simulink model "MECROKA_TWR_B"  (R2017b)
settings: Solver=FixedStepDiscrete  StartTime=0.0  StopTime=inf  RelTol=1e-3  EnableMultiTasking=on
InitFcn:
  | % BLDC-data
  | num_pol_pairs = 7
  | res_period = 5000;
  | res_pwm   = 2^8;
  | 
  | wheel_radius=0.033;
  | axle_length=0.2;
undefined symbols (not defined in the file): DiscIntNeverNeededParam
libraries: MecRoKa_SFunction_Library x18, arduinolib x12, simulink x5, simulink_extras x2
(part 1 of 2)
settings Model: ExtModeTrigDuration=2  Creator=Bitsch  LastModifiedBy=Lenovo
settings DataIOCC: LimitDataPoints=on  InspectSignalLogs=on
settings OptimizationCC: LifeSpan=1  MaxStackSize=64
settings DebuggingCC: UnderspecifiedInitializationDetection=Classic  MergeDetectMultiDrivingBlocksExec=none  ParameterPrecisionLossMsg=none  AllowSymbolicDim=off  SFUnexpectedBacktrackingDiag=warning  SFNoUnconditionalDefaultTransitionDiag=warning  SFExecutionAtInitializationDiag=none
settings HardwareCC: ProdBitPerPointer=32  ProdBitPerSizeT=32  ProdBitPerPtrDiffT=32  ProdLargestAtomicInteger=Long  ProdLargestAtomicFloat=Double  ProdWordSize=32  ProdHWDeviceType=ARM Compatible->ARM Cortex  UseEmbeddedCoderFeatures=off  UseSimulinkCoderFeatures=off
settings ModelReferenceCC: PropagateSignalLabelsOutOfModel=off
settings SFSimCC: MATLABDynamicMemAlloc=off
settings RTWCC: SystemTargetFile=ert.tlc  HardwareBoard=Arduino Due  TLCOptions=-aInlineSetEventsForThisBaseRateFcn=TLC_FALSE -aSuppressMultiTaskScheduler=TLC_FALSE -aRateBasedStepFcn=1  TemplateMakefile=ert_default_tmf  Toolchain=Arduino ARM  BuildConfiguration=Faster Runs
settings CodeAppCC: StateflowObjectComments=on
settings ERTTargetCC: MultiwordLength=2048  ERTCustomFileBanners=off  SupportContinuousTime=on  SupportNonInlinedSFcns=on  RemoveResetFunc=off  ModelStepFunctionPrototypeControlCompliant=off  ConvertIfToSwitch=off  SuppressUnreachableDefaultCases=off
settings ConfigComp: CovMetricSettings=dw  CovHtmlReporting=on  CovSaveCumulativeToWorkspaceVar=on  CovSaveSingleToWorkspaceVar=on  CovExternalEMLEnable=off

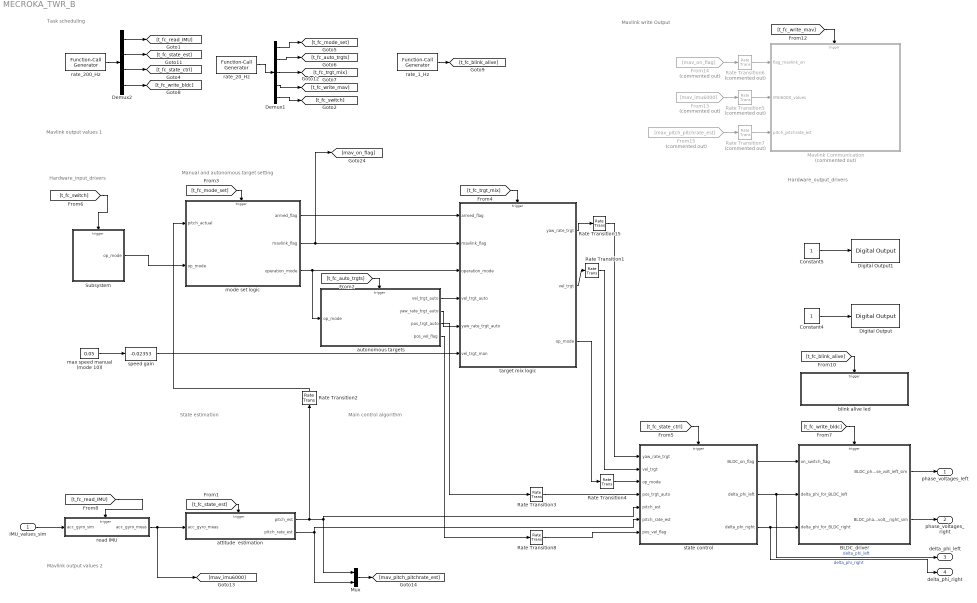
== system MECROKA_TWR_B ==
  note: Mavlink write Output
  note: Mavlink output values 2
  note: Mavlink output values 1
  note: Task scheduling
  note: Manual and autonomous target setting
  note: State estimation
  note: Hardware_output_drivers
  note: Hardware_input_drivers
  note: Main control algorithm
  IMU_values_sim : Inport  OutDataTypeStr=int32  PortDimensions=6
  BLDC_driver : Subsystem  TreatAsAtomicUnit=on
  Constant4 : Constant
  Constant5 : Constant
  Demux1 : Demux  Outputs=5
  Demux2 : Demux
  Digital Output : arduinolib/Digital Output  pinNumber=22  blockPlatform=arduino
  Digital Output1 : arduinolib/Digital Output  pinNumber=24  blockPlatform=arduino
  From13 : From  Commented=on  GotoTag=mav_imu6000
  From14 : From  Commented=on  GotoTag=mav_on_flag
  From15 : From  Commented=on  GotoTag=mav_pitch_pitchrate_est
  Mavlink Communication : Stateflow chart  Commented=on  TreatAsAtomicUnit=on
  Mux : Mux  Inputs=2
  Rate Transition{1..4,8,15} (6 alike) : RateTransition  OutPortSampleTimeOpt=Inherit  OutPortSampleTime=0.01
  Rate Transition5 : RateTransition  Commented=on  OutPortSampleTimeOpt=Inherit  OutPortSampleTime=0.01
  Rate Transition6 : RateTransition  Commented=on  OutPortSampleTimeOpt=Inherit  OutPortSampleTime=0.01
  Rate Transition7 : RateTransition  Commented=on  OutPortSampleTimeOpt=Inherit  OutPortSampleTime=0.01
  Subsystem : Subsystem
  attitude  estimation : Stateflow chart  TreatAsAtomicUnit=on
  autonomous targets : Stateflow chart  TreatAsAtomicUnit=on
  blink alive led : Subsystem  TreatAsAtomicUnit=on
  max speed manual (mode 10)l : Constant  Value=0.05  OutDataTypeStr=double
  mode set logic : Stateflow chart  TreatAsAtomicUnit=on
  rate_1_Hz : simulink/Ports & Subsystems/Function-Call Generator  sample_time=1  numberOfIterations=1
  rate_200_Hz : simulink/Ports & Subsystems/Function-Call Generator  sample_time=0.005  numberOfIterations=1
  rate_20_Hz : simulink/Ports & Subsystems/Function-Call Generator  sample_time=0.05  numberOfIterations=1
  read IMU : Subsystem  TreatAsAtomicUnit=on
  speed gain : simulink/Math Operations/Slider Gain  gain=-0.02353  low=-1  high=1
  state control : Stateflow chart  TreatAsAtomicUnit=on
  target mix logic : Stateflow chart  TreatAsAtomicUnit=on
  phase_voltages_left : Outport
  phase_voltages_right : Outport  Port=2
  delta_phi_left : Outport  Port=3  OutDataTypeStr=double
  delta_phi_right : Outport  Port=4  OutDataTypeStr=double
  wires:
  rate_1_Hz/1 -> [t_fc_blink_alive]
  Rate Transition4/1 -> state control/3(op_mode)
  rate_200_Hz/1 -> Demux2/1
  mode set logic/1(armed_flag) -> target mix logic/1(armed_flag)
  [t_fc_auto_trgts] -> autonomous targets/Trigger
  [t_fc_read_IMU] -> read IMU/Trigger
  Demux2/3 -> [t_fc_state_ctrl]
  rate_20_Hz/1 -> Demux1/1
  target mix logic/3(op_mode) -> Rate Transition4/1
  Demux2/2 -> [t_fc_state_est]
  Rate Transition15/1 -> state control/1(yaw_rate_trgt)
  attitude  estimation/1(pitch_est) -> Rate Transition2/1, Mux/1, state control/5(pitch_est)
  Demux2/1 -> [t_fc_read_IMU]
  [t_fc_state_est] -> attitude  estimation/Trigger
  mode set logic/3(operation_mode) -> autonomous targets/1(op_mode), target mix logic/3(operation_mode)
  [t_fc_state_ctrl] -> state control/Trigger
  Demux2/4 -> [t_fc_write_bldc]
  [t_fc_blink_alive] -> blink alive led/Trigger
  target mix logic/1(yaw_rate_trgt) -> Rate Transition15/1
  target mix logic/2(vel_trgt) -> Rate Transition1/1
  autonomous targets/2(yaw_rate_trgt_auto) -> target mix logic/5(yaw_rate_trgt_auto)
  [t_fc_mode_set] -> mode set logic/Trigger
  read IMU/1(acc_gyro_meas) -> [mav_imu6000], attitude  estimation/1(acc_gyro_meas)
  autonomous targets/1(vel_trgt_auto) -> target mix logic/4(vel_trgt_auto)
  Rate Transition1/1 -> state control/2(vel_trgt)
  IMU_values_sim/1 -> read IMU/1(acc_gyro_sim)
  mode set logic/2(mavlink_flag) -> [mav_on_flag], target mix logic/2(mavlink_flag)
  [t_fc_trgt_mix] -> target mix logic/Trigger
  attitude  estimation/2(pitch_rate_est) -> Mux/2, state control/6(pitch_rate_est)
  [t_fc_write_mav] -> Mavlink Communication/Trigger
  From13/1 -> Rate Transition5/1
  Rate Transition5/1 -> Mavlink Communication/2(IMU6000_values)
  From14/1 -> Rate Transition6/1
  Rate Transition6/1 -> Mavlink Communication/1(flag_mavlink_on)
  Mux/1 -> [mav_pitch_pitchrate_est]
  Rate Transition7/1 -> Mavlink Communication/3(pitch_pitchrate_est)
  From15/1 -> Rate Transition7/1
  state control/2(delta_phi_left) -> delta_phi_left/1, BLDC_driver/2(delta_phi_for_BLDC_left)  "delta_phi_left"
  state control/3(delta_phi_right) -> delta_phi_right/1, BLDC_driver/3(delta_phi_for_BLDC_right)  "delta_phi_right"
  Demux1/1 -> [t_fc_mode_set]
  Demux1/2 -> [t_fc_auto_trgts]
  Demux1/3 -> [t_fc_trgt_mix]
  Demux1/4 -> [t_fc_write_mav]
  [t_fc_write_bldc] -> BLDC_driver/Trigger
  BLDC_driver/1(BLDC_phase_volt_left_sim) -> phase_voltages_left/1
  BLDC_driver/2(BLDC_phase_volt__right_sim) -> phase_voltages_right/1
  speed gain/1 -> target mix logic/6(vel_trgt_man)
  max speed manual (mode 10)l/1 -> speed gain/1
  Rate Transition2/1 -> mode set logic/1(pitch_actual)
  state control/1(BLDC_on_flag) -> BLDC_driver/1(on_switch_flag)
  Constant4/1 -> Digital Output/1
  Constant5/1 -> Digital Output1/1
  autonomous targets/3(pos_trgt_auto) -> Rate Transition3/1
  Rate Transition3/1 -> state control/4(pos_trgt_auto)
  autonomous targets/4(pos_vel_flag) -> Rate Transition8/1
  Rate Transition8/1 -> state control/7(pos_vel_flag)
  Subsystem/1(op_mode) -> mode set logic/2(op_mode)
  Demux1/5 -> [t_fc_switch]
  [t_fc_switch] -> Subsystem/Trigger

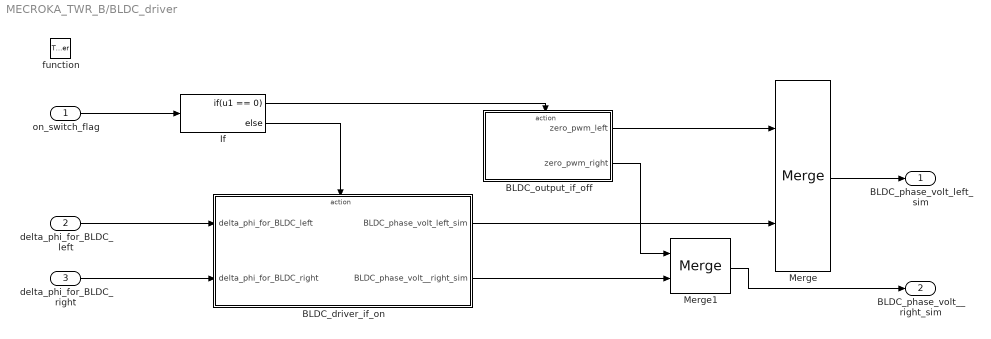
== system MECROKA_TWR_B/BLDC_driver ==
  on_switch_flag : Inport  OutDataTypeStr=boolean  PortDimensions=1
  delta_phi_for_BLDC_left : Inport  Port=2  OutDataTypeStr=double  PortDimensions=1
  delta_phi_for_BLDC_right : Inport  Port=3  OutDataTypeStr=double  PortDimensions=1
  function : TriggerPort  TriggerType=function-call  VariantControl=(inherit)
  BLDC_driver_if_on : Subsystem  TreatAsAtomicUnit=on
  BLDC_output_if_off : Subsystem  TreatAsAtomicUnit=on
  If : If  IfExpression=u1 == 0
  Merge : Merge
  Merge1 : Merge
  BLDC_phase_volt_left_sim : Outport  OutDataTypeStr=uint16  PortDimensions=3
  BLDC_phase_volt__right_sim : Outport  Port=2  OutDataTypeStr=uint16  PortDimensions=3
  wires:
  delta_phi_for_BLDC_right/1 -> BLDC_driver_if_on/2(delta_phi_for_BLDC_right)
  on_switch_flag/1 -> If/1
  BLDC_output_if_off/1(zero_pwm_left) -> Merge/1
  Merge/1 -> BLDC_phase_volt_left_sim/1
  If/1 -> BLDC_output_if_off/Action
  Merge1/1 -> BLDC_phase_volt__right_sim/1
  BLDC_driver_if_on/1(BLDC_phase_volt_left_sim) -> Merge/2
  If/2 -> BLDC_driver_if_on/Action
  BLDC_driver_if_on/2(BLDC_phase_volt__right_sim) -> Merge1/2
  BLDC_output_if_off/2(zero_pwm_right) -> Merge1/1
  delta_phi_for_BLDC_left/1 -> BLDC_driver_if_on/1(delta_phi_for_BLDC_left)

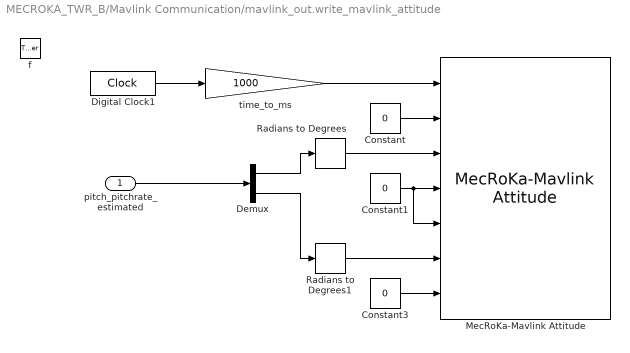
== system MECROKA_TWR_B/Mavlink Communication/mavlink_out.write_mavlink_attitude ==
  pitch_pitchrate_estimated : Inport  OutDataTypeStr=double  PortDimensions=2
  f : TriggerPort  TriggerType=function-call  VariantControl=(inherit)
      settings: CopyFcn=Stateflow.SLINSF.SimulinkMan.removeBlockPreDeleteFcn  PreDeleteFcn=Stateflow.SLINSF.SimulinkMan.unsafePredeleteFcn
  Constant : Constant  Value=0  OutDataTypeStr=double
  Constant1 : Constant  Value=0  OutDataTypeStr=double
  Constant3 : Constant  Value=0  OutDataTypeStr=double
  Demux : Demux  Outputs=2
  Digital Clock1 : DigitalClock  SampleTime=-1
  MecRoKa-Mavlink Attitude : MecRoKa_SFunction_Library/Arduino-Blocks/Mavlink-Library /MecRoKa-Mavlink Attitude  serialPort=0  baudRate=115200  sys_id=2  comp_id=MAV_COMP_ID_ALL
      settings: SourceProductName=MecRoKa_SFunction-Library
  Radians to Degrees : simulink_extras/Transformations/Radians to Degrees
  Radians to Degrees1 : simulink_extras/Transformations/Radians to Degrees
  time_to_ms : Gain  Gain=1000  OutDataTypeStr=uint32
  wires:
  Constant/1 -> MecRoKa-Mavlink Attitude/2
  time_to_ms/1 -> MecRoKa-Mavlink Attitude/1
  Digital Clock1/1 -> time_to_ms/1
  Constant1/1 -> MecRoKa-Mavlink Attitude/5, MecRoKa-Mavlink Attitude/4
  pitch_pitchrate_estimated/1 -> Demux/1
  Demux/1 -> Radians to Degrees/1
  Demux/2 -> Radians to Degrees1/1
  Constant3/1 -> MecRoKa-Mavlink Attitude/7
  Radians to Degrees/1 -> MecRoKa-Mavlink Attitude/3
  Radians to Degrees1/1 -> MecRoKa-Mavlink Attitude/6

== system MECROKA_TWR_B/Mavlink Communication/mavlink_out.write_mavlink_heartbeat ==
  f : TriggerPort  TriggerType=function-call  VariantControl=(inherit)
      settings: CopyFcn=Stateflow.SLINSF.SimulinkMan.removeBlockPreDeleteFcn  PreDeleteFcn=Stateflow.SLINSF.SimulinkMan.unsafePredeleteFcn
  MecRoKa-Mavlink Heartbeat : MecRoKa_SFunction_Library/Arduino-Blocks/Mavlink-Library /MecRoKa-Mavlink Heartbeat  serialPort=0  baudRate=115200  sys_id=2  comp_id=MAV_COMP_ID_ALL  types=MAV_TYPE_GENERIC  autopilot=MAV_AUTOPILOT_GENERIC  base_mode=MAV_MODE_MANUAL_ARMED  custom_mode_m=1  system_status=MAV_STATE_ACTIVE
      settings: SourceProductName=MecRoKa_SFunction-Library

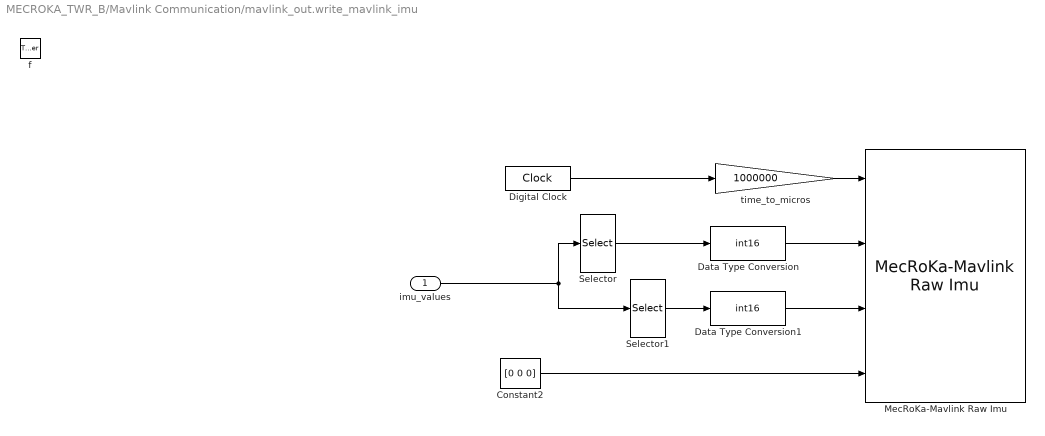
== system MECROKA_TWR_B/Mavlink Communication/mavlink_out.write_mavlink_imu ==
  imu_values : Inport  OutDataTypeStr=int32  PortDimensions=6
  f : TriggerPort  TriggerType=function-call  VariantControl=(inherit)
      settings: CopyFcn=Stateflow.SLINSF.SimulinkMan.removeBlockPreDeleteFcn  PreDeleteFcn=Stateflow.SLINSF.SimulinkMan.unsafePredeleteFcn
  Constant2 : Constant  Value=[0 0 0]  OutDataTypeStr=int16
  Data Type Conversion : DataTypeConversion  OutDataTypeStr=int16
  Data Type Conversion1 : DataTypeConversion  OutDataTypeStr=int16
  Digital Clock : DigitalClock  SampleTime=-1
  MecRoKa-Mavlink Raw Imu : MecRoKa_SFunction_Library/Arduino-Blocks/Mavlink-Library /MecRoKa-Mavlink Raw Imu  serialPort=0  baudRate=115200  sys_id=2  comp_id=MAV_COMP_ID_ALL
      settings: SourceProductName=MecRoKa_SFunction-Library
  Selector : Selector  InputPortWidth=6  IndexOptions=Index vector (dialog)  Indices=[1 2 3]  OutputSizes=1
  Selector1 : Selector  InputPortWidth=6  IndexOptions=Index vector (dialog)  Indices=[4 5 6]  OutputSizes=1
  time_to_micros : Gain  Gain=1000000  OutDataTypeStr=uint32
  wires:
  Data Type Conversion/1 -> MecRoKa-Mavlink Raw Imu/2
  Selector/1 -> Data Type Conversion/1
  Data Type Conversion1/1 -> MecRoKa-Mavlink Raw Imu/3
  Selector1/1 -> Data Type Conversion1/1
  Constant2/1 -> MecRoKa-Mavlink Raw Imu/4
  time_to_micros/1 -> MecRoKa-Mavlink Raw Imu/1
  Digital Clock/1 -> time_to_micros/1
  imu_values/1 -> Selector/1, Selector1/1

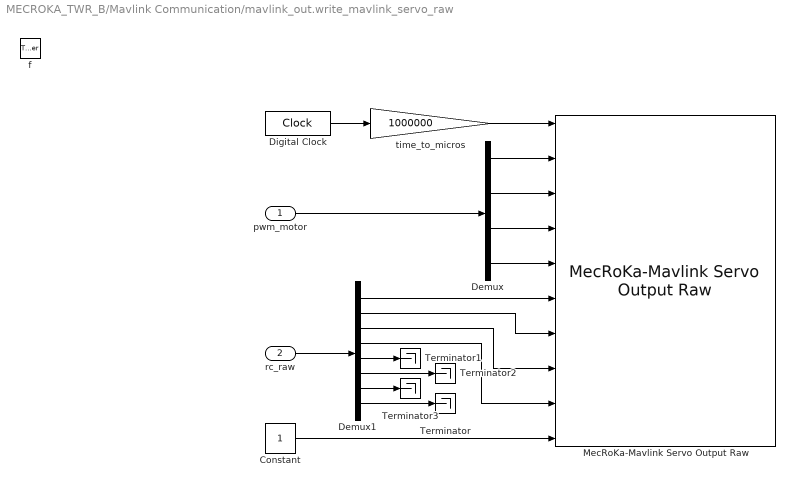
== system MECROKA_TWR_B/Mavlink Communication/mavlink_out.write_mavlink_servo_raw ==
  pwm_motor : Inport  OutDataTypeStr=uint16  PortDimensions=4
  rc_raw : Inport  Port=2  OutDataTypeStr=uint16  PortDimensions=8
  f : TriggerPort  TriggerType=function-call  VariantControl=(inherit)
      settings: CopyFcn=Stateflow.SLINSF.SimulinkMan.removeBlockPreDeleteFcn  PreDeleteFcn=Stateflow.SLINSF.SimulinkMan.unsafePredeleteFcn
  Constant : Constant  OutDataTypeStr=uint8
  Demux : Demux
  Demux1 : Demux  Outputs=8
  Digital Clock : DigitalClock  SampleTime=-1
  MecRoKa-Mavlink Servo Output Raw : MecRoKa_SFunction_Library/Mavlink-Library /MecRoKa-Mavlink Servo Output Raw  serialPort=2  baudRate=57600  sys_id=1  comp_id=MAV_COMP_ID_ALL
      settings: SourceProductName=MecRoKa_SFunction-Library
  Terminator{,1..3} (4 alike) : Terminator
  time_to_micros : Gain  Gain=1000000  OutDataTypeStr=uint32
  wires:
  Demux/1 -> MecRoKa-Mavlink Servo Output Raw/2
  Demux/2 -> MecRoKa-Mavlink Servo Output Raw/3
  Demux/3 -> MecRoKa-Mavlink Servo Output Raw/4
  Demux/4 -> MecRoKa-Mavlink Servo Output Raw/5
  time_to_micros/1 -> MecRoKa-Mavlink Servo Output Raw/1
  Digital Clock/1 -> time_to_micros/1
  Demux1/1 -> MecRoKa-Mavlink Servo Output Raw/6
  Demux1/2 -> MecRoKa-Mavlink Servo Output Raw/7
  Demux1/3 -> MecRoKa-Mavlink Servo Output Raw/8
  Demux1/4 -> MecRoKa-Mavlink Servo Output Raw/9
  pwm_motor/1 -> Demux/1
  Demux1/8 -> Terminator/1
  Demux1/7 -> Terminator3/1
  Demux1/6 -> Terminator2/1
  Demux1/5 -> Terminator1/1
  rc_raw/1 -> Demux1/1
  Constant/1 -> MecRoKa-Mavlink Servo Output Raw/10

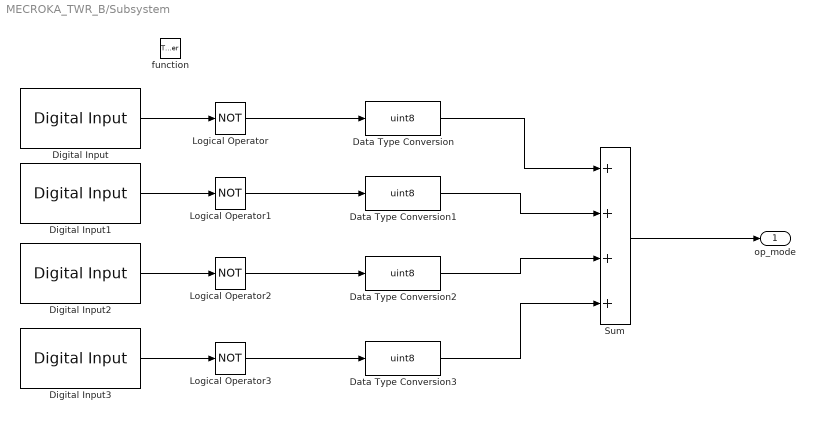
== system MECROKA_TWR_B/Subsystem ==
  function : TriggerPort  TriggerType=function-call  VariantControl=Variant
  Data Type Conversion{,1..3} (4 alike) : DataTypeConversion  OutDataTypeStr=uint8
  Digital Input : arduinolib/Digital Input  pinNumber=9  sampleTime=-1  blockPlatform=arduino
      settings: SourceProductName=Simulink Support Package for Arduino Hardware
  Digital Input1 : arduinolib/Digital Input  pinNumber=10  sampleTime=-1  blockPlatform=arduino
      settings: SourceProductName=Simulink Support Package for Arduino Hardware
  Digital Input2 : arduinolib/Digital Input  pinNumber=11  sampleTime=-1  blockPlatform=arduino
      settings: SourceProductName=Simulink Support Package for Arduino Hardware
  Digital Input3 : arduinolib/Digital Input  pinNumber=12  sampleTime=-1  blockPlatform=arduino
      settings: SourceProductName=Simulink Support Package for Arduino Hardware
  Logical Operator{,1..3} (4 alike) : Logic  Operator=NOT  AllPortsSameDT=off  OutDataTypeStr=boolean
  Sum : Sum  Inputs=++++
  op_mode : Outport
  wires:
  Digital Input1/1 -> Logical Operator1/1
  Digital Input/1 -> Logical Operator/1
  Data Type Conversion/1 -> Sum/1
  Sum/1 -> op_mode/1
  Data Type Conversion1/1 -> Sum/2
  Digital Input2/1 -> Logical Operator2/1
  Digital Input3/1 -> Logical Operator3/1
  Data Type Conversion2/1 -> Sum/3
  Data Type Conversion3/1 -> Sum/4
  Logical Operator/1 -> Data Type Conversion/1
  Logical Operator1/1 -> Data Type Conversion1/1
  Logical Operator2/1 -> Data Type Conversion2/1
  Logical Operator3/1 -> Data Type Conversion3/1

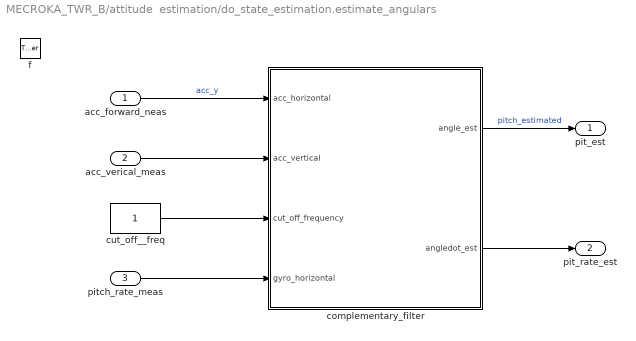
== system MECROKA_TWR_B/attitude  estimation/do_state_estimation.estimate_angulars ==
  acc_forward_neas : Inport  OutDataTypeStr=int32  PortDimensions=1
  acc_verical_meas : Inport  Port=2  OutDataTypeStr=int32  PortDimensions=1
  pitch_rate_meas : Inport  Port=3  OutDataTypeStr=int32  PortDimensions=1
  f : TriggerPort  TriggerType=function-call  VariantControl=(inherit)
      settings: CopyFcn=Stateflow.SLINSF.SimulinkMan.removeBlockPreDeleteFcn  PreDeleteFcn=Stateflow.SLINSF.SimulinkMan.unsafePredeleteFcn
  complementary_filter : Subsystem
  cut_off__freq : Constant
  pit_est : Outport  OutDataTypeStr=double
  pit_rate_est : Outport  Port=2  OutDataTypeStr=double
  wires:
  acc_verical_meas/1 -> complementary_filter/2(acc_vertical)
  pitch_rate_meas/1 -> complementary_filter/4(gyro_horizontal)
  acc_forward_neas/1 -> complementary_filter/1(acc_horizontal)  "acc_y"
  cut_off__freq/1 -> complementary_filter/3(cut_off_frequency)
  complementary_filter/2(angledot_est) -> pit_rate_est/1
  complementary_filter/1(angle_est) -> pit_est/1  "pitch_estimated"

== system MECROKA_TWR_B/blink alive led ==
  function : TriggerPort  TriggerType=function-call  VariantControl=(inherit)
  MecRoKa-TogglePin : MecRoKa_SFunction_Library/Arduino-Blocks/Arduino-Library/MecRoKa-TogglePin  pinNumber=13
      settings: SourceProductName=MecRoKa_SFunction-Library

== system MECROKA_TWR_B/read IMU ==
  acc_gyro_sim : Inport  OutDataTypeStr=int32  PortDimensions=6
  function : TriggerPort  TriggerType=function-call  VariantControl=(inherit)
  Constant : Constant  OutDataTypeStr=int32
  Demux : Demux  Outputs=2
  MecRoKa-IMU6000 : MecRoKa_SFunction_Library/Arduino-Blocks/Sensor-Library/MecRoKa-IMU6000  selectWire=0
      settings: SourceProductName=MecRoKa_SFunction-Library
  Mux : Mux  Inputs=2
  Terminator : Terminator
  acc_gyro_meas : Outport  OutDataTypeStr=int32  PortDimensions=6
  wires:
  acc_gyro_sim/1 -> Demux/1
  Mux/1 -> acc_gyro_meas/1
  Demux/1 -> MecRoKa-IMU6000/1
  Demux/2 -> MecRoKa-IMU6000/2
  MecRoKa-IMU6000/1 -> Mux/1
  MecRoKa-IMU6000/2 -> Mux/2
  MecRoKa-IMU6000/3 -> Terminator/1
  Constant/1 -> MecRoKa-IMU6000/3

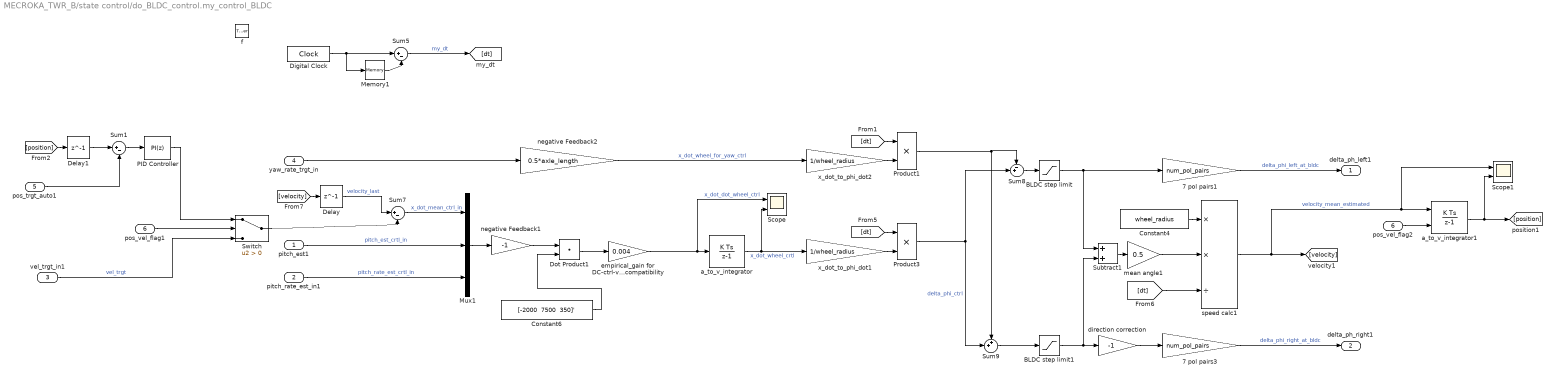
== system MECROKA_TWR_B/state control/do_BLDC_control.my_control_BLDC ==
  pitch_est1 : Inport  OutDataTypeStr=double  PortDimensions=1
  pitch_rate_est_in1 : Inport  Port=2  OutDataTypeStr=double  PortDimensions=1
  vel_trgt_in1 : Inport  Port=3  OutDataTypeStr=double  PortDimensions=1
  yaw_rate_trgt_in : Inport  Port=4  OutDataTypeStr=double  PortDimensions=1
  pos_trgt_auto1 : Inport  Port=5  OutDataTypeStr=double  PortDimensions=1
  pos_vel_flag1 : Inport  Port=6  OutDataTypeStr=double  PortDimensions=1
  f : TriggerPort  TriggerType=function-call  VariantControl=(inherit)
      settings: CopyFcn=Stateflow.SLINSF.SimulinkMan.removeBlockPreDeleteFcn  PreDeleteFcn=Stateflow.SLINSF.SimulinkMan.unsafePredeleteFcn
  7 pol pairs1 : Gain  Gain=num_pol_pairs
  7 pol pairs3 : Gain  Gain=num_pol_pairs
  BLDC step limit : Saturate  UpperLimit=0.11  LowerLimit=-0.11
  BLDC step limit1 : Saturate  UpperLimit=0.11  LowerLimit=-0.11
  Constant4 : Constant  Value=wheel_radius
  Constant6 : Constant  Value="[-2000  7500  350]'"  OutDataTypeStr=double
  Delay : Delay  DelayLength=1  InitialCondition=0
  Delay1 : Delay  DelayLength=1  InitialCondition=0
  Digital Clock : DigitalClock  SampleTime=-1
  Dot Product1 : DotProduct  InputSameDT=on  OutDataTypeStr=Inherit: Inherit via internal rule
  Memory1 : Memory  InitialCondition=-0.008  InheritSampleTime=on  LinearizeAsDelay=on
  Mux1 : Mux  Inputs=3
  PID Controller : simulink/Continuous/PID Controller  Controller=PI  TimeDomain=Discrete-time  SampleTime=-1  IntegratorMethod=Forward Euler  FilterMethod=Forward Euler  Form=Parallel  UseFilter=off  ControllerParametersSource=internal  P=-1.7  I=-1.2  D=-0.2  N=100  InitialConditionSource=internal  InitialConditionForIntegrator=-0.1  InitialConditionForFilter=0  ExternalReset=none  LimitOutput=on  UpperSaturationLimit=0.7  LowerSaturationLimit=-0.7  LinearizeAsGain=on  AntiWindupMode=clamping  Kb=1  TrackingMode=off  Kt=1  PParamMin=[]  PParamMax=[]  IParamMin=[]  IParamMax=[]  DParamMin=[]  DParamMax=[]  NParamMin=[]  NParamMax=[]  KbParamMin=[]  KbParamMax=[]  KtParamMin=[]  KtParamMax=[]  POutMin=[]  POutMax=[]  IOutMin=[]  IOutMax=[]  DOutMin=[]  DOutMax=[]  NOutMin=[]  NOutMax=[]  KbOutMin=[]  KbOutMax=[]  KtOutMin=[]  KtOutMax=[]  IntegratorOutMin=[]  IntegratorOutMax=[]  FilterOutMin=[]  FilterOutMax=[]  SumOutMin=[]  SumOutMax=[]  SumI1OutMin=[]  SumI1OutMax=[]  SumI2OutMin=[]  SumI2OutMax=[]  SumI3OutMin=[]  SumI3OutMax=[]  SumDOutMin=[]  SumDOutMax=[]  SaturationOutMin=[]  SaturationOutMax=[]  IntegratorContinuousStateAttributes=''  IntegratorStateMustResolveToSignalObject=off  IntegratorRTWStateStorageClass=Auto  FilterContinuousStateAttributes=''  FilterStateMustResolveToSignalObject=off  FilterRTWStateStorageClass=Auto  DifferentiatorICPrevScaledInput=0  DifferentiatorOutMin=[]  DifferentiatorOutMax=[]  InitialConditionSetting=State (most efficient)  FilterDiffOutCoefMin=[]  FilterDiffOutCoefMax=[]  SumDenOutMin=[]  SumDenOutMax=[]  SumNumOutMin=[]  SumNumOutMax=[]  ReciprocalOutMin=[]  ReciprocalOutMax=[]  DivideOutMin=[]  DivideOutMax=[]  TunerSelectOption=Transfer Function Based (PID Tuner App)
  Product1 : Product
  Product3 : Product
  Scope : Scope  NumInputPorts=2
  Scope1 : Scope  NumInputPorts=2
  Subtract1 : Sum
  Sum1 : Sum  Inputs=|+-
  Sum5 : Sum  Inputs=|+-
  Sum7 : Sum  Inputs=|+-
  Sum8 : Sum  Inputs=-+|
  Sum9 : Sum  Inputs=++|
  Switch : Switch  Criteria=u2 > Threshold
  a_to_v_integrator : DiscreteIntegrator  SampleTime=-1  LimitOutput=on  UpperSaturationLimit=1  LowerSaturationLimit=-1  ICPrevOutput=DiscIntNeverNeededParam  ICPrevScaledInput=DiscIntNeverNeededParam
  a_to_v_integrator1 : DiscreteIntegrator  ExternalReset=rising  SampleTime=-1  UpperSaturationLimit=0  LowerSaturationLimit=0  ICPrevOutput=DiscIntNeverNeededParam  ICPrevScaledInput=DiscIntNeverNeededParam
  direction correction : Gain  Gain=-1
  empirical_gain for DC-ctrl-values-compatibility : Gain  Gain=0.004
  mean angle1 : Gain  Gain=0.5  OutDataTypeStr=double
  negative Feedback1 : Gain  Gain=-1
  negative Feedback2 : Gain  Gain=0.5*axle_length
  pos_vel_flag2 : InportShadow  Port=6  OutDataTypeStr=double  PortDimensions=1
  speed calc1 : Product  Inputs=**/
  x_dot_to_phi_dot1 : Gain  Gain=1/wheel_radius
  x_dot_to_phi_dot2 : Gain  Gain=1/wheel_radius
  delta_ph_left1 : Outport  OutDataTypeStr=double  PortDimensions=1
  delta_ph_right1 : Outport  Port=2  OutDataTypeStr=double  PortDimensions=1
  wires:
  Sum5/1 -> [dt]  "my_dt"
  Digital Clock/1 -> Memory1/1, Sum5/1
  Memory1/1 -> Sum5/2
  Mux1/1 -> negative Feedback1/1
  negative Feedback1/1 -> Dot Product1/1
  Sum7/1 -> Mux1/1  "x_dot_mean_ctrl_in"
  Constant6/1 -> Dot Product1/2
  yaw_rate_trgt_in/1 -> negative Feedback2/1
  Product1/1 -> Sum8/1, Sum9/1
  [velocity] -> Delay/1
  vel_trgt_in1/1 -> Switch/3  "vel_trgt"
  pitch_est1/1 -> Mux1/2  "pitch_est_crtl_in"
  pitch_rate_est_in1/1 -> Mux1/3  "pitch_rate_est_crtl_in"
  empirical_gain for DC-ctrl-values-compatibility/1 -> Scope/1, a_to_v_integrator/1  "x_dot_dot_wheel_ctrl"
  Dot Product1/1 -> empirical_gain for DC-ctrl-values-compatibility/1
  x_dot_to_phi_dot1/1 -> Product3/2
  Product3/1 -> Sum9/2, Sum8/2  "delta_phi_ctrl"
  [dt] -> Product3/1
  Sum8/1 -> BLDC step limit/1
  Sum9/1 -> BLDC step limit1/1
  [dt] -> speed calc1/3
  BLDC step limit1/1 -> Subtract1/2, direction correction/1
  Subtract1/1 -> mean angle1/1
  mean angle1/1 -> speed calc1/2
  Constant4/1 -> speed calc1/1
  speed calc1/1 -> Scope1/1, a_to_v_integrator1/1, [velocity]  "velocity_mean_estimated"
  Delay/1 -> Sum7/1  "velocity_last"
  BLDC step limit/1 -> 7 pol pairs1/1, Subtract1/1
  7 pol pairs1/1 -> delta_ph_left1/1  "delta_phi_left_at_bldc"
  direction correction/1 -> 7 pol pairs3/1
  7 pol pairs3/1 -> delta_ph_right1/1  "delta_phi_right_at_bldc"
  a_to_v_integrator/1 -> Scope/2, x_dot_to_phi_dot1/1  "x_dot_wheel_crtl"
  x_dot_to_phi_dot2/1 -> Product1/2
  [dt] -> Product1/1
  negative Feedback2/1 -> x_dot_to_phi_dot2/1  "x_dot_wheel_for_yaw_ctrl"
  a_to_v_integrator1/1 -> Scope1/2, [position]
  [position] -> Delay1/1
  Delay1/1 -> Sum1/1
  Switch/1 -> Sum7/2
  pos_trgt_auto1/1 -> Sum1/2
  Sum1/1 -> PID Controller/1
  PID Controller/1 -> Switch/1
  pos_vel_flag1/1 -> Switch/2
  pos_vel_flag2/1 -> a_to_v_integrator1/2

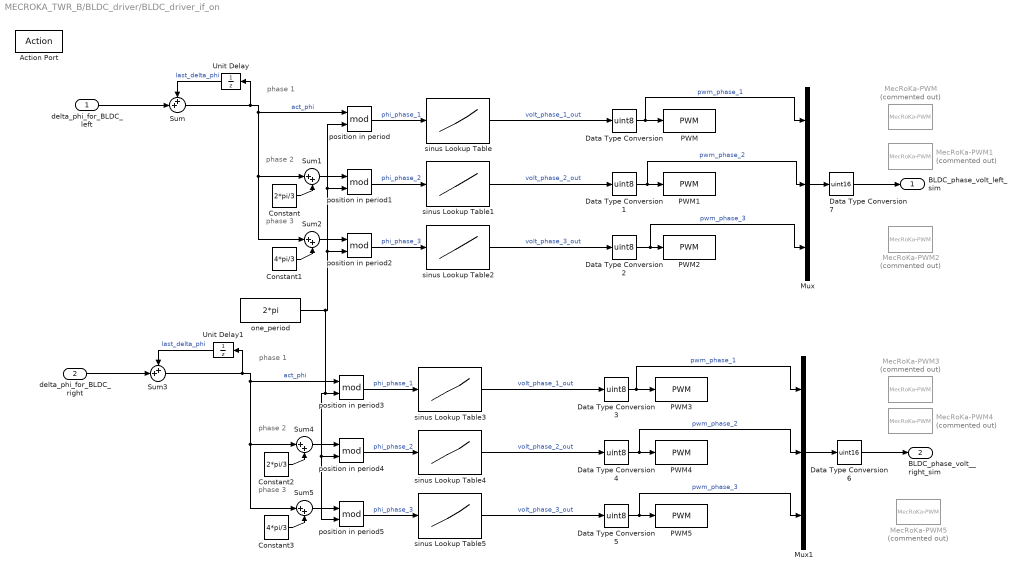
== system MECROKA_TWR_B/BLDC_driver/BLDC_driver_if_on ==
  note: phase 3
  note: phase 2
  note: phase 1
  note: phase 3
  note: phase 2
  note: phase 1
  delta_phi_for_BLDC_left : Inport  OutDataTypeStr=double  PortDimensions=1
  delta_phi_for_BLDC_right : Inport  Port=2  OutDataTypeStr=double  PortDimensions=1
  Action Port : ActionPort  ActionType=else
  Constant : Constant  Value=2*pi/3
  Constant1 : Constant  Value=4*pi/3
  Constant2 : Constant  Value=2*pi/3
  Constant3 : Constant  Value=4*pi/3
  Data Type Conversion{,1..5} (6 alike) : DataTypeConversion  OutDataTypeStr=uint8
  Data Type Conversion6 : DataTypeConversion  OutDataTypeStr=uint16
  Data Type Conversion7 : DataTypeConversion  OutDataTypeStr=uint16
  MecRoKa-PWM : MecRoKa_SFunction_Library/Arduino-Blocks/Arduino-Library/MecRoKa-PWM  Commented=on  pinNumber=6
      settings: SourceProductName=MecRoKa_SFunction-Library
  MecRoKa-PWM1 : MecRoKa_SFunction_Library/Arduino-Blocks/Arduino-Library/MecRoKa-PWM  Commented=on  pinNumber=8
      settings: SourceProductName=MecRoKa_SFunction-Library
  MecRoKa-PWM2 : MecRoKa_SFunction_Library/Arduino-Blocks/Arduino-Library/MecRoKa-PWM  Commented=on  pinNumber=7
      settings: SourceProductName=MecRoKa_SFunction-Library
  MecRoKa-PWM3 : MecRoKa_SFunction_Library/Arduino-Blocks/Arduino-Library/MecRoKa-PWM  Commented=on  pinNumber=3
      settings: SourceProductName=MecRoKa_SFunction-Library
  MecRoKa-PWM4 : MecRoKa_SFunction_Library/Arduino-Blocks/Arduino-Library/MecRoKa-PWM  Commented=on  pinNumber=4
      settings: SourceProductName=MecRoKa_SFunction-Library
  MecRoKa-PWM5 : MecRoKa_SFunction_Library/Arduino-Blocks/Arduino-Library/MecRoKa-PWM  Commented=on  pinNumber=5
      settings: SourceProductName=MecRoKa_SFunction-Library
  Mux : Mux  Inputs=3
  Mux1 : Mux  Inputs=3
  PWM : arduinolib/PWM  pinNumber=6  blockPlatform=arduino
  PWM1 : arduinolib/PWM  pinNumber=7  blockPlatform=arduino
  PWM2 : arduinolib/PWM  pinNumber=8  blockPlatform=arduino
  PWM3 : arduinolib/PWM  pinNumber=3  blockPlatform=arduino
  PWM4 : arduinolib/PWM  pinNumber=4  blockPlatform=arduino
  PWM5 : arduinolib/PWM  pinNumber=5  blockPlatform=arduino
  Sum : Sum  Inputs=++|
  Sum{1..2,4..5} (4 alike) : Sum  Inputs=|++
  Sum3 : Sum  Inputs=++|
  Unit Delay : UnitDelay  SampleTime=-1
  Unit Delay1 : UnitDelay  SampleTime=-1
  one_period : Constant  Value=2*pi
  position in period{,1..5} (6 alike) : Math  Operator=mod  SaturateOnIntegerOverflow=on
  sinus Lookup Table : Lookup_n-D  NumberOfTableDimensions=1  BreakpointsSpecification=Even spacing  BreakpointsForDimension1=[0:0.25:2*pi]  BreakpointsForDimension2=[0:0.25:2*pi]  BreakpointsForDimension3=[0:0.25:2*pi]  BreakpointsForDimension1FirstPoint=0  BreakpointsForDimension1Spacing=2*pi/res_period  BreakpointsForDimension2Spacing=0.25  BreakpointsForDimension3Spacing=0.25  BeginIndexSearchUsingPreviousIndexResult=on  Table=(res_pwm/2-1)*sin([0:2*pi/res_period:2*pi])+(res_pwm/2-1)  InterpMethod=Nearest  ExtrapMethod=Cubic spline  InternalRulePriority=Speed  OutDataTypeStr=uint16  RndMeth=Simplest  InputSameDT=on
  sinus Lookup Table{1..2,4..5} (4 alike) : Lookup_n-D  NumberOfTableDimensions=1  BreakpointsSpecification=Even spacing  BreakpointsForDimension1=[0:0.25:2*pi]  BreakpointsForDimension2=[0:0.25:2*pi]  BreakpointsForDimension3=[0:0.25:2*pi]  BreakpointsForDimension1FirstPoint=0  BreakpointsForDimension1Spacing=2*pi/res_period  BreakpointsForDimension2Spacing=0.25  BreakpointsForDimension3Spacing=0.25  BeginIndexSearchUsingPreviousIndexResult=on  Table=(res_pwm/2-1)*sin([0:2*pi/res_period:2*pi]) +(res_pwm/2-1)  InterpMethod=Nearest  ExtrapMethod=Cubic spline  InternalRulePriority=Speed  OutDataTypeStr=uint16  RndMeth=Simplest  InputSameDT=on
  sinus Lookup Table3 : Lookup_n-D  NumberOfTableDimensions=1  BreakpointsSpecification=Even spacing  BreakpointsForDimension1=[0:0.25:2*pi]  BreakpointsForDimension2=[0:0.25:2*pi]  BreakpointsForDimension3=[0:0.25:2*pi]  BreakpointsForDimension1FirstPoint=0  BreakpointsForDimension1Spacing=2*pi/res_period  BreakpointsForDimension2Spacing=0.25  BreakpointsForDimension3Spacing=0.25  BeginIndexSearchUsingPreviousIndexResult=on  Table=(res_pwm/2-1)*sin([0:2*pi/res_period:2*pi])+(res_pwm/2-1)  InterpMethod=Nearest  ExtrapMethod=Cubic spline  InternalRulePriority=Speed  OutDataTypeStr=uint16  RndMeth=Simplest  InputSameDT=on
  BLDC_phase_volt_left_sim : Outport  OutDataTypeStr=uint16  PortDimensions=3
  BLDC_phase_volt__right_sim : Outport  Port=2  OutDataTypeStr=uint16  PortDimensions=3
  wires:
  sinus Lookup Table/1 -> Data Type Conversion/1  "volt_phase_1_out"
  Unit Delay/1 -> Sum/1  "last_delta_phi"
  Sum/1 -> position in period/1, Sum2/1, Sum1/1, Unit Delay/1  "act_phi"
  Sum1/1 -> position in period1/1
  Sum2/1 -> position in period2/1
  Constant/1 -> Sum1/2
  position in period1/1 -> sinus Lookup Table1/1  "phi_phase_2"
  position in period2/1 -> sinus Lookup Table2/1  "phi_phase_3"
  sinus Lookup Table1/1 -> Data Type Conversion1/1  "volt_phase_2_out"
  sinus Lookup Table2/1 -> Data Type Conversion2/1  "volt_phase_3_out"
  Constant1/1 -> Sum2/2
  position in period/1 -> sinus Lookup Table/1  "phi_phase_1"
  Mux/1 -> Data Type Conversion7/1
  Data Type Conversion/1 -> Mux/1, PWM/1  "pwm_phase_1"
  Data Type Conversion1/1 -> Mux/2, PWM1/1  "pwm_phase_2"
  Data Type Conversion2/1 -> Mux/3, PWM2/1  "pwm_phase_3"
  delta_phi_for_BLDC_left/1 -> Sum/2
  one_period/1 -> position in period5/2, position in period4/2, position in period3/2, position in period/2, position in period1/2, position in period2/2
  Unit Delay1/1 -> Sum3/1  "last_delta_phi"
  Sum3/1 -> position in period3/1, Sum5/1, Sum4/1, Unit Delay1/1  "act_phi"
  Sum4/1 -> position in period4/1
  Sum5/1 -> position in period5/1
  Constant2/1 -> Sum4/2
  position in period4/1 -> sinus Lookup Table4/1  "phi_phase_2"
  position in period5/1 -> sinus Lookup Table5/1  "phi_phase_3"
  Constant3/1 -> Sum5/2
  position in period3/1 -> sinus Lookup Table3/1  "phi_phase_1"
  Mux1/1 -> Data Type Conversion6/1
  Data Type Conversion3/1 -> Mux1/1, PWM3/1  "pwm_phase_1"
  Data Type Conversion4/1 -> Mux1/2, PWM4/1  "pwm_phase_2"
  Data Type Conversion5/1 -> Mux1/3, PWM5/1  "pwm_phase_3"
  sinus Lookup Table3/1 -> Data Type Conversion3/1  "volt_phase_1_out"
  sinus Lookup Table4/1 -> Data Type Conversion4/1  "volt_phase_2_out"
  sinus Lookup Table5/1 -> Data Type Conversion5/1  "volt_phase_3_out"
  delta_phi_for_BLDC_right/1 -> Sum3/2
  Data Type Conversion7/1 -> BLDC_phase_volt_left_sim/1
  Data Type Conversion6/1 -> BLDC_phase_volt__right_sim/1

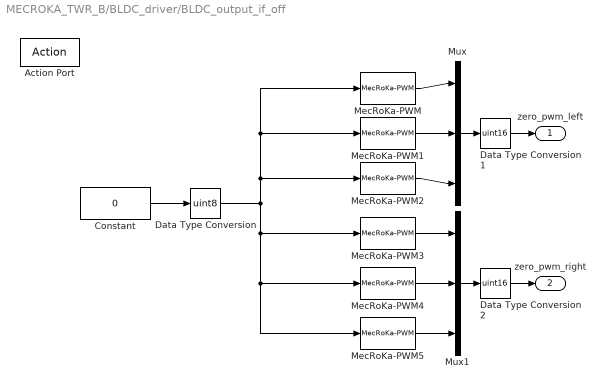
== system MECROKA_TWR_B/BLDC_driver/BLDC_output_if_off ==
  Action Port : ActionPort  ActionType=then
  Constant : Constant  Value=0  OutDataTypeStr=uint16
  Data Type Conversion : DataTypeConversion  OutDataTypeStr=uint8
  Data Type Conversion1 : DataTypeConversion  OutDataTypeStr=uint16
  Data Type Conversion2 : DataTypeConversion  OutDataTypeStr=uint16
  MecRoKa-PWM : MecRoKa_SFunction_Library/Arduino-Blocks/Arduino-Library/MecRoKa-PWM  pinNumber=6
      settings: SourceProductName=MecRoKa_SFunction-Library
  MecRoKa-PWM1 : MecRoKa_SFunction_Library/Arduino-Blocks/Arduino-Library/MecRoKa-PWM  pinNumber=8
      settings: SourceProductName=MecRoKa_SFunction-Library
  MecRoKa-PWM2 : MecRoKa_SFunction_Library/Arduino-Blocks/Arduino-Library/MecRoKa-PWM  pinNumber=7
      settings: SourceProductName=MecRoKa_SFunction-Library
  MecRoKa-PWM3 : MecRoKa_SFunction_Library/Arduino-Blocks/Arduino-Library/MecRoKa-PWM  pinNumber=3
      settings: SourceProductName=MecRoKa_SFunction-Library
  MecRoKa-PWM4 : MecRoKa_SFunction_Library/Arduino-Blocks/Arduino-Library/MecRoKa-PWM  pinNumber=4
      settings: SourceProductName=MecRoKa_SFunction-Library
  MecRoKa-PWM5 : MecRoKa_SFunction_Library/Arduino-Blocks/Arduino-Library/MecRoKa-PWM  pinNumber=5
      settings: SourceProductName=MecRoKa_SFunction-Library
  Mux : Mux  Inputs=3
  Mux1 : Mux  Inputs=3
  zero_pwm_left : Outport
  zero_pwm_right : Outport  Port=2
  wires:
  Constant/1 -> Data Type Conversion/1
  Data Type Conversion/1 -> MecRoKa-PWM5/1, MecRoKa-PWM4/1, MecRoKa-PWM3/1, MecRoKa-PWM1/1, MecRoKa-PWM/1, MecRoKa-PWM2/1
  MecRoKa-PWM/1 -> Mux/1
  MecRoKa-PWM1/1 -> Mux/2
  MecRoKa-PWM2/1 -> Mux/3
  MecRoKa-PWM3/1 -> Mux1/1
  MecRoKa-PWM4/1 -> Mux1/2
  MecRoKa-PWM5/1 -> Mux1/3
  Mux1/1 -> Data Type Conversion2/1
  Mux/1 -> Data Type Conversion1/1
  Data Type Conversion1/1 -> zero_pwm_left/1
  Data Type Conversion2/1 -> zero_pwm_right/1

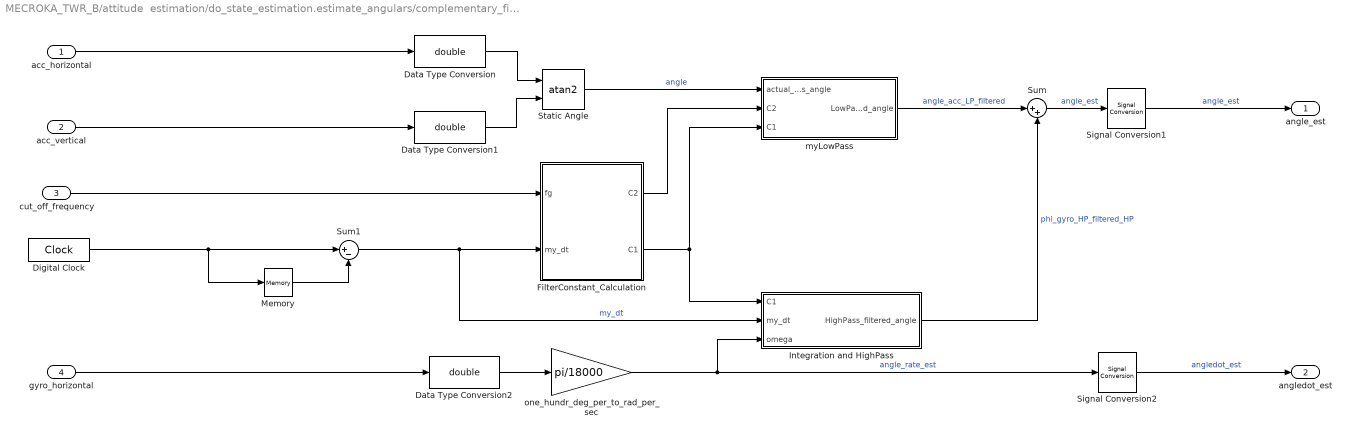
== system MECROKA_TWR_B/attitude  estimation/do_state_estimation.estimate_angulars/complementary_filter ==
  acc_horizontal : Inport
  acc_vertical : Inport  Port=2
  cut_off_frequency : Inport  Port=3
  gyro_horizontal : Inport  Port=4
  Data Type Conversion : DataTypeConversion  OutDataTypeStr=double
  Data Type Conversion1 : DataTypeConversion  OutDataTypeStr=double
  Data Type Conversion2 : DataTypeConversion  OutDataTypeStr=double
  Digital Clock : DigitalClock  SampleTime=-1
  FilterConstant_Calculation : Subsystem
  Integration and HighPass : Subsystem
  Memory : Memory  InheritSampleTime=on  LinearizeAsDelay=on
  Signal Conversion1 : SignalConversion  OverrideOpt=off
  Signal Conversion2 : SignalConversion  OverrideOpt=off
  Static Angle : Trigonometry  Operator=atan2  OutputSignalType=real
  Sum : Sum  Inputs=|++
  Sum1 : Sum  Inputs=|+-
  myLowPass : Subsystem  TreatAsAtomicUnit=on
  one_hundr_deg_per_to_rad_per_sec : Gain  Gain=pi/18000
  angle_est : Outport  PortDimensions=1
  angledot_est : Outport  Port=2  PortDimensions=1
  wires:
  FilterConstant_Calculation/2(C1) -> myLowPass/3(C1), Integration and HighPass/1(C1)
  myLowPass/1(LowPass_filtered_angle) -> Sum/1  "angle_acc_LP_filtered"
  cut_off_frequency/1 -> FilterConstant_Calculation/1(fg)
  one_hundr_deg_per_to_rad_per_sec/1 -> Signal Conversion2/1, Integration and HighPass/3(omega)  "angle_rate_est"
  Static Angle/1 -> myLowPass/1(actual_meas_angle)  "angle"
  FilterConstant_Calculation/1(C2) -> myLowPass/2(C2)
  Sum/1 -> Signal Conversion1/1  "angle_est"
  Integration and HighPass/1(HighPass_filtered_angle) -> Sum/2  "phi_gyro_HP_filtered_HP"
  Data Type Conversion2/1 -> one_hundr_deg_per_to_rad_per_sec/1
  Signal Conversion2/1 -> angledot_est/1  "angledot_est"
  Data Type Conversion/1 -> Static Angle/1
  Data Type Conversion1/1 -> Static Angle/2
  Sum1/1 -> Integration and HighPass/2(my_dt), FilterConstant_Calculation/2(my_dt)  "my_dt"
  Signal Conversion1/1 -> angle_est/1  "angle_est"
  gyro_horizontal/1 -> Data Type Conversion2/1
  acc_vertical/1 -> Data Type Conversion1/1
  acc_horizontal/1 -> Data Type Conversion/1
  Digital Clock/1 -> Memory/1, Sum1/1
  Memory/1 -> Sum1/2

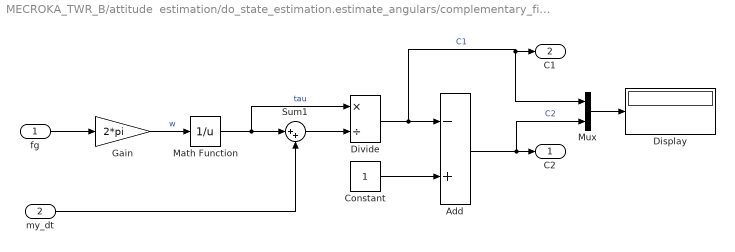
== system MECROKA_TWR_B/attitude  estimation/do_state_estimation.estimate_angulars/complementary_filter/FilterConstant_Calculation ==
  fg : Inport
  my_dt : Inport  Port=2
  Add : Sum  Inputs=-+
  Constant : Constant
  Display : Display
      settings: Decimation=3
  Divide : Product  Inputs=*/
  Gain : Gain  Gain=2*pi
  Math Function : Math  Operator=reciprocal  SaturateOnIntegerOverflow=on
  Mux : Mux  Inputs=2
  Sum1 : Sum  Inputs=|++
  C2 : Outport
  C1 : Outport  Port=2
  wires:
  Math Function/1 -> Divide/1, Sum1/1  "tau"
  Gain/1 -> Math Function/1  "w"
  Sum1/1 -> Divide/2
  fg/1 -> Gain/1
  my_dt/1 -> Sum1/2
  Divide/1 -> Mux/1, C1/1, Add/1  "C1"
  Constant/1 -> Add/2
  Add/1 -> Mux/2, C2/1  "C2"
  Mux/1 -> Display/1

== system MECROKA_TWR_B/attitude  estimation/do_state_estimation.estimate_angulars/complementary_filter/Integration and HighPass ==
  C1 : Inport
  my_dt : Inport  Port=2
  omega : Inport  Port=3
  Memory : Memory  InheritSampleTime=on
  Product : Product  RndMeth=Zero
  Product1 : Product  RndMeth=Zero
  Sum1 : Sum  Inputs=|++
  HighPass_filtered_angle : Outport
  wires:
  Memory/1 -> Sum1/2
  Product1/1 -> Memory/1, HighPass_filtered_angle/1
  Product/1 -> Sum1/1
  omega/1 -> Product/2
  my_dt/1 -> Product/1
  Sum1/1 -> Product1/2
  C1/1 -> Product1/1

== system MECROKA_TWR_B/attitude  estimation/do_state_estimation.estimate_angulars/complementary_filter/myLowPass ==
  actual_meas_angle : Inport  OutDataTypeStr=double
  C2 : Inport  Port=2
  C1 : Inport  Port=3
  Memory : Memory  InitialCondition=0*pi/180  InheritSampleTime=on
  Product : Product  RndMeth=Zero
  Product1 : Product  RndMeth=Zero
  Sum1 : Sum  Inputs=|++
  LowPass_filtered_angle : Outport
  wires:
  actual_meas_angle/1 -> Product1/1
  Sum1/1 -> Memory/1, LowPass_filtered_angle/1
  Product/1 -> Sum1/2
  Product1/1 -> Sum1/1
  C1/1 -> Product/2
  Memory/1 -> Product/1
  C2/1 -> Product1/2

== stateflow chart MECROKA_TWR_B/state control ==
  state system_off
    en, du: delta_phi_left   = double(0.0);
    en, du: delta_phi_right = double(0.0);
    en, du: BLDC_on_flag = false;
  state do_BLDC_control
    en, du: BLDC_on_flag = true;
    en, du : [delta_phi_left, delta_phi_right]=my_control_BLDC(pitch_est, pitch_rate_est, vel_trgt, yaw_rate_trgt,pos_trgt_auto, pos_vel_flag);
    state [delta_ph_left1,delta_ph_right1] = my_control_BLDC(pitch_est1,pitch_rate_est_in1,vel_trgt_in1,yaw_rate_trgt_in,pos_trgt_auto1,pos_vel_flag1) [function]
  (default) -> system_off
  system_off -> do_BLDC_control : [op_mode ~= 0 ]
  do_BLDC_control -> system_off : [op_mode == 0 ]
  data: pitch_est1 function_input double size=1; pitch_rate_est_in1 function_input double size=1; vel_trgt_in1 function_input double size=1; yaw_rate_trgt_in function_input double size=1; delta_ph_left1 function_output double size=1; delta_ph_right1 function_output double size=1; pos_trgt_auto1 function_input double size=1; pos_vel_flag1 function_input double size=1; BLDC_on_flag output boolean; yaw_rate_trgt input double size=1; vel_trgt input double size=1; op_mode input uint8 size=1; pos_trgt_auto input double size=1; pitch_est input double size=1; pitch_rate_est input double size=1; delta_phi_left output double size=1; delta_phi_right output double size=1; pos_vel_flag input double size=1
  events: t_fc_state_ctrl input FUNCTION_CALL_EVENT

== stateflow chart MECROKA_TWR_B/target mix logic ==
  state disarmed
    en, du: op_mode = op_mode;
    en, du: vel_trgt = 0;
    en, du: yaw_rate_trgt  = 0;
  state armed
    en, du: op_mode = operation_mode;
    en, du: yaw_rate_trgt  = yaw_rate_trgt_auto;
    state autonomous
      en, du: vel_trgt   = vel_trgt_auto;
    state manual
      en, du: vel_trgt   = vel_trgt_man;
    (default) -> (junction 18)
    (junction 18) -> autonomous [order 2]
    autonomous -> armed
    (junction 18) -> manual [order 1] : [operation_mode == 10]
    manual -> armed
  (default) -> (junction 15)
  (junction 15) -> armed [order 1] : [armed_flag == true]
  (junction 15) -> disarmed [order 2]
  disarmed -> armed : [armed_flag == true]
  armed -> disarmed : [armed_flag == false]
  data: yaw_rate_trgt output double size=1; vel_trgt output double size=1; armed_flag input boolean size=1; mavlink_flag input boolean size=1; operation_mode input uint8 size=1; vel_trgt_auto input double size=1; yaw_rate_trgt_auto input double size=1; op_mode output uint8 size=1; vel_trgt_man input double size=1
  events: t_fc_trgt_mix_logic input FUNCTION_CALL_EVENT

== stateflow chart MECROKA_TWR_B/attitude  estimation ==
  state do_state_estimation
    en: [pitch_est, pitch_rate_est]           = estimate_angulars(acc_gyro_meas(2), acc_gyro_meas(3), acc_gyro_meas(4));
    state [pit_est, pit_rate_est] = estimate_angulars(acc_forward_neas, acc_verical_meas, pitch_rate_meas) [function]
  (default) -> do_state_estimation
  do_state_estimation -> do_state_estimation
  data: acc_forward_neas function_input int32 size=1; acc_verical_meas function_input int32 size=1; pit_est function_output double; pitch_rate_meas function_input int32 size=1; pit_rate_est function_output double; pitch_est output double size=1; pitch_rate_est output double size=1; acc_gyro_meas input int32 size=6
  events: t_fc_state_est input FUNCTION_CALL_EVENT

== stateflow chart MECROKA_TWR_B/mode set logic ==
  state set_actual_mode
    state set_autonomous_targets
      en: armed_flag = true;
      en: mavlink_flag = true;
      en: operation_mode = op_mode;
    state swich_off_if_high_pitch
      en: operation_mode = uint8(0);
    (default) -> (junction 22)
    (junction 22) -> swich_off_if_high_pitch [order 1] : [abs(pitch_actual)>50*2*pi/360]
    (junction 22) -> set_autonomous_targets [order 2]
    swich_off_if_high_pitch -> set_actual_mode
    set_autonomous_targets -> set_actual_mode
  (default) -> set_actual_mode
  data: armed_flag output boolean size=1; mavlink_flag output boolean size=1; operation_mode output uint8 size=1; pitch_actual input double size=1; op_mode input uint8 size=1
  events: t_fc_mode_set_logic input FUNCTION_CALL_EVENT
